simulink model "BiasedWireOpenLoop"  (R2021b)
settings: Solver=VariableStepAuto  StartTime=0.0  StopTime=50  RelTol=1e-3
values from neighbouring files (symbols this model uses):
  A = 4.9e-8    (= 4.9e-08)    [init.m]
  b_s = 0.5    [init.m]
  I = 2.7e-6    (= 2.7e-06)    [init.m]
  k_s = 0.0018    [init.m]
  r = 7.5e-3    (= 0.0075)    [init.m]
settings Model: Creator=Raj Shah  LastModifiedBy=Raj Shah

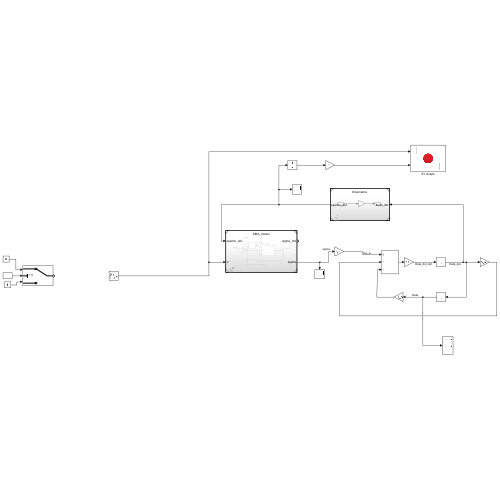
[thumbnail: Simulink's stored preview of the top-level diagram]
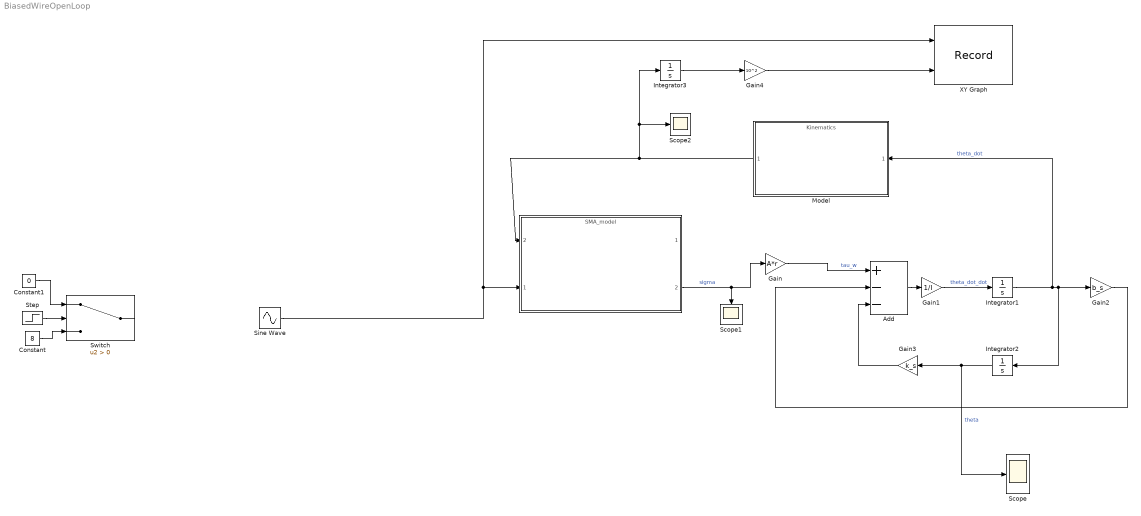
== system BiasedWireOpenLoop ==
  " " : ModelReference  ModelNameDialog=SMA_model.slx  SimulationMode=Normal  ModelReferenceVersion=1.40
      settings: PortSchema="{\"entries\":[{\"content\":{\"sides\":[{\"content\":{\"connectorIds\":[\"In2\",\"In1\"]},\"type\":\"ConnectorPlacement.EquallySpacedRectSide\",\"uuid\":\"608ed256-bf4a-4468-aaa6-41a0901fe41c\"},{\"content\":{\"connectorIds\":[\"Out1\",\"Out2\"],\"side\":\"RIGHT\"},\"type\":\"ConnectorPlacement.EquallySpacedRectSide\",\"uuid\":\"ea926bb8-49f4-4647-b1e1-2602f3a83e1c\"},{\"content\":{\"connectorIds\":[],\"side\":\"TOP\"},\"type\":\"ConnectorPlacement.EquallySpacedRectSide\",\"uuid\":\"2990464a-009d-4220-9d5a-e567065e0ad2\"}]},\"type\":\"ConnectorPlacement.EquallySpacedConnector\",\"uuid\":\"de33bc14-3798-4fc1-9250-22d458448bf7\"}],\"packageUris\":[\"http://schema.mathworks.com/mf0/Connector/R2020b\"],\"version\":\"1.0\"}"
  Add : Sum  Inputs=+--
  Constant : Constant  Value=8
  Constant1 : Constant  Value=0
  Gain : Gain  Gain=A*r
  Gain1 : Gain  Gain=1/I
  Gain2 : Gain  Gain=b_s
  Gain3 : Gain  Gain=k_s
  Gain4 : Gain  Gain=10^2
  Integrator1 : Integrator
  Integrator2 : Integrator
  Integrator3 : Integrator
  Model : ModelReference  ModelNameDialog=Kinematics.slx  SimulationMode=Normal  ModelReferenceVersion=1.1
  Scope : Scope
  Scope1 : Scope
  Scope2 : Scope
  Sine Wave : Sin  Amplitude=8  Frequency=0.1  SampleTime=0
  Step : Step  Time=10  SampleTime=0
  Switch : Switch  Criteria=u2 > Threshold
  XY Graph : Record  FileSettingsInternal="{\"entries\":[{\"content\":{\"excelSettings\":{\"content\":{},\"type\":\"Streamout.ExcelSettings\"}},\"type\":\"Streamout.FileSettingStorage\",\"uuid\":\"df0d4909-8a03-4eec-9ded-e912c76b0fc2\"}],\"packageUris\":[\"http://schema.mathworks.com/mf0/streamout_blocks/R2020a\"],\"version\":\"1.0\"}"  Layout=[1 1]  SignalsInternal="{\"entries\":[{\"content\":{\"signals\":[{\"content\":{\"blockPath\":[\"BiasedWireOpenLoop/XY Graph\"],\"channel\":[],\"dimensions\":[1],\"domain\":\"BiasedWireOpenLoop/XY Graph\",\"lineColor\":\"#a2142f\",\"plots\":[1],\"port\":1,\"sid\":[\"\"],\"signalID\":45774,\"signalName\":\"Sine Wave\"},\"type\":\"RecordBlkView.Signal\",\"uuid\":\"8f5b2ed7-6832-4e79-b1a9-0139660d3cd2\"},{\"content\":{\"blockPath\":[\"BiasedWireOpenLoop/XY Graph\"],\"channel\":[],\"dimensions\":[1],\"domain\":\"BiasedWireOpenLoop/XY Graph\",\"lineColor\":\"#139fff\",\"plots\":[1],\"port\":2,\"sid\":[\"\"],\"signalID\":45778,\"signalName\":\"Gain4\"},\"type\":\"RecordBlkView.Signal\",\"uuid\":\"76f42208-3520-41aa-b0d5-bad6a64ed8c0\"}]},\"type\":\"RecordBlkView.InputSignals\",\"uuid\":\"aabf0cd8-72d3-4628-ac82-332a183cecd0\"}],\"packageUris\":[\"http://schema.mathworks.com/mf0/streamout_blocks/R2020a\"],\"version\":\"1.0\"}"  CompatibilityTag=XY
  wires:
  Model/1 -> Scope2/1, Integrator3/1, " "/2
  Sine Wave/1 -> XY Graph/1, " "/1
  " "/2 -> Scope1/1, Gain/1  "sigma"
  Gain/1 -> Add/1  "tau_w"
  Add/1 -> Gain1/1
  Gain1/1 -> Integrator1/1  "theta_dot_dot"
  Integrator1/1 -> Integrator2/1, Gain2/1, Model/1  "theta_dot"
  Gain2/1 -> Add/2
  Gain3/1 -> Add/3
  Integrator2/1 -> Scope/1, Gain3/1  "theta"
  Integrator3/1 -> Gain4/1
  Gain4/1 -> XY Graph/2
  Step/1 -> Switch/2
  Constant/1 -> Switch/3
  Constant1/1 -> Switch/1
